simulink model "oltf2"  (R2025b)
settings: Solver=FixedStepAuto  StartTime=0.0  StopTime=10.0  FixedStep=1e-3  RelTol=1e-3
values from neighbouring files (symbols this model uses):
  A = 1    [rlelog2.m]    (also in rlelog6_.m)
  den_ac = [1 0.8608 5.3159942 0.108928 0.0529]    [rlelog6_.m]
  Kp = 3.5    [rlelog6_.m]
  num_ac = [3.476 3.1708072 0.0896237936]    [rlelog6_.m]
  R = 0.725    [rlelog2.m]    (also in rlelog6_.m)
  w = freqs(i)    [rlelog2.m]    (also in rlelog6_.m = omega(i))
settings Model: Creator=t0900  LastModifiedBy=t0900

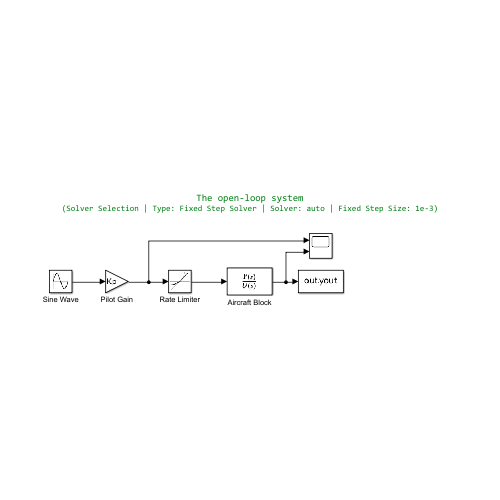
[thumbnail: Simulink's stored preview of the top-level diagram]
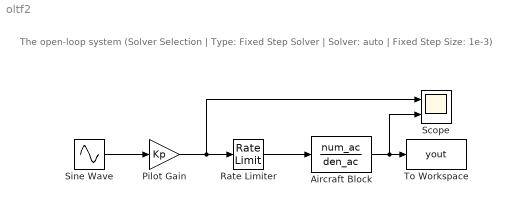
== system oltf2 ==
  note: The open-loop system
      | (Solver Selection | Type: Fixed Step Solver | Solver: auto | Fixed Step Size: 1e-3)
  Aircraft Block : TransferFcn  Numerator=num_ac  Denominator=den_ac
  Pilot Gain : Gain  Gain=Kp
  Rate Limiter : RateLimiter  RisingSlewLimit=R  FallingSlewLimit=-R
  Scope : Scope  NumInputPorts=2
      settings: ActiveDisplayYMinimum=-85.522211262942463  ActiveDisplayYMaximum=90.1589722845847  YLabel=Pilot Command
  Sine Wave : Sin  Amplitude=A  Frequency=w  SampleTime=0
  To Workspace : ToWorkspace  VariableName=yout  SaveFormat=Timeseries  SampleTime=-1
  wires:
  Sine Wave/1 -> Pilot Gain/1
  Rate Limiter/1 -> Aircraft Block/1
  Pilot Gain/1 -> Scope/1, Rate Limiter/1
  Aircraft Block/1 -> To Workspace/1, Scope/2
